simulink model "sampleModel1601_2"  (R2023a)
settings: Solver=VariableStepAuto  StartTime=0.0  StopTime=10.0  RelTol=1e-3
libraries: hdlsllib x2, simulink x1
settings Model: Creator=user1  LastModifiedBy=user1

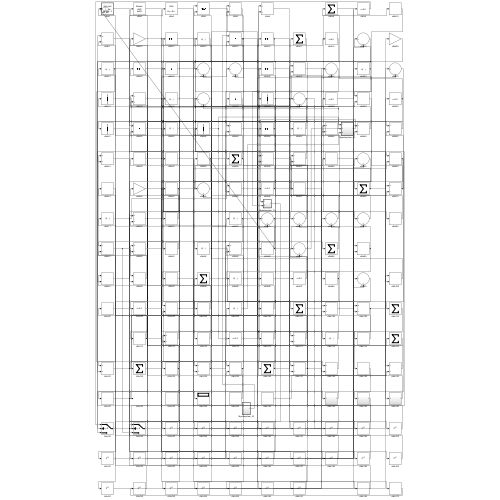
[thumbnail: Simulink's stored preview of the top-level diagram]
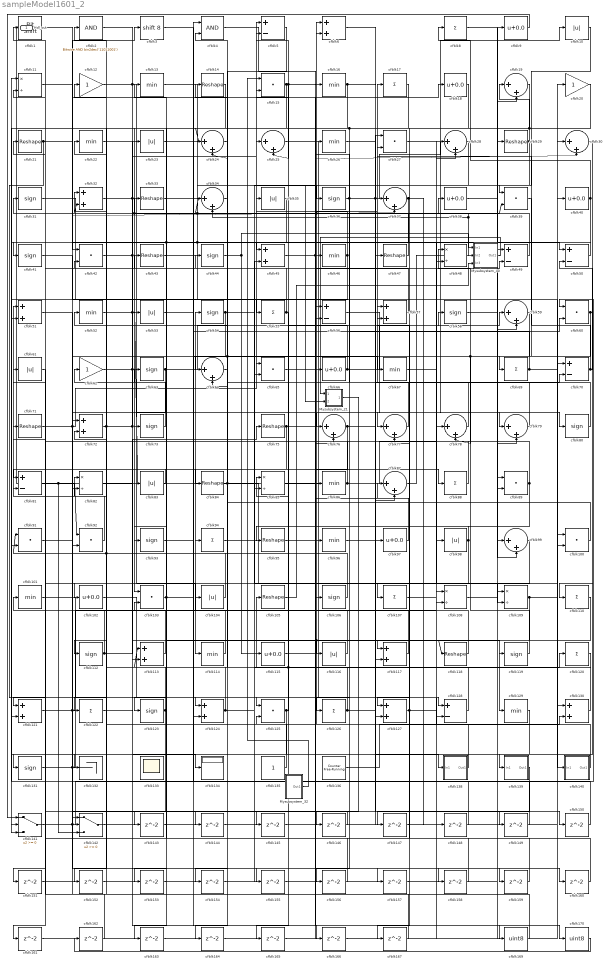
== system sampleModel1601_2 ==
  Mysubsystem_21 : Subsystem  TreatAsAtomicUnit=on  RTWFcnName=Mysubsystem_21
      settings: RTWFcnNameOpts=User specified  RTWFileNameOpts=Use function name
  Mysubsystem_32 : Subsystem  TreatAsAtomicUnit=on  RTWFcnName=Mysubsystem_32
      settings: RTWFcnNameOpts=User specified  RTWFileNameOpts=Use function name
  Mysubsystem_40 : Subsystem  TreatAsAtomicUnit=on  RTWFcnName=Mysubsystem_40
      settings: RTWFcnNameOpts=User specified  RTWFileNameOpts=Use function name
  cfblk1 : hdlsllib/Logic and Bit Operations/Bit Shift  mode=Shift Left Logical  N=0
  cfblk{10,23,35,53,61,83,98,104,116} (9 alike) : Abs  OutDataTypeStr=uint8  SaturateOnIntegerOverflow=off
  cfblk{15,27,39,42,60,65,89,91..92,100,103,125} (12 alike) : DotProduct  OutDataTypeStr=uint8
  cfblk{13,16,22,26,46,52,67,86,96,101,114,129} (12 alike) : MinMax  OutDataTypeStr=uint8
  cfblk{9,18,38,40,66,97,102,115} (8 alike) : Bias  Bias=0.0  SaturateOnIntegerOverflow=off
  cfblk{14,21,29,33,43,47,71,75,84,95,105,118} (12 alike) : Reshape
  cfblk{31,36,41,44,54,58,63,73,80,93,106,112,119,123,131} (15 alike) : Signum
  cfblk{8,17,55,69,88,94,107,110,120,122,126} (11 alike) : Sum  Inputs=+  OutDataTypeStr=uint8
  cfblk{11,48,82,85,108..109} (6 alike) : Product  Inputs=*/  OutDataTypeStr=uint8  RndMeth=Zero  SaturateOnIntegerOverflow=on
  cfblk{6,32,45,51,57,72,113,117,121,124,127,130} (12 alike) : Sum  OutDataTypeStr=uint8
  cfblk12 : Gain  OutDataTypeStr=uint8
  cfblk{5,49..50,56,70,81,128} (7 alike) : Sum  Inputs=+-  OutDataTypeStr=uint8
  cfblk132 : Terminator
  cfblk133 : Scope
      settings: Floating=on
  cfblk134 : Display
  cfblk135 : Constant  OutDataTypeStr=uint8  SampleTime=-1
  cfblk136 : hdlsllib/Sources/Counter Free-Running  NumBits=16  tsamp=-1
  cfblk138 : Subsystem
      settings: LibrarySourceBlock=|
      | hdlsllib/Ports &
      | Subsystems/Subsystem
  cfblk139 : Subsystem
      settings: LibrarySourceBlock=|
      | hdlsllib/Ports &
      | Subsystems/Subsystem
  cfblk140 : Subsystem
      settings: LibrarySourceBlock=|
      | hdlsllib/Ports &
      | Subsystems/Subsystem
  cfblk141 : Switch  OutDataTypeStr=uint8  SaturateOnIntegerOverflow=off  InputSameDT=off
  cfblk142 : Switch  OutDataTypeStr=uint8  SaturateOnIntegerOverflow=off  InputSameDT=off
  cfblk{143..167} (25 alike) : Delay  SampleTime=1
  cfblk169 : DataTypeConversion  OutDataTypeStr=uint8  SaturateOnIntegerOverflow=off  RndMeth=Floor
  cfblk170 : DataTypeConversion  OutDataTypeStr=uint8  SaturateOnIntegerOverflow=off  RndMeth=Floor
  cfblk{19,24..25,28,30,34,37,59,64,76..79,87,99} (15 alike) : Sum  Inputs=|++  OutDataTypeStr=uint8
  cfblk2 : simulink/Logic and Bit Operations/Bitwise Operator  logicop=AND  UseBitMask=on  BitMask=bin2dec('11011001')  BitMaskRealWorld=Stored Integer
      settings: LibrarySourceBlock=|
      | hdlsllib/Logic and Bit
      | Operations/Bitwise
      | Operator
  cfblk20 : Gain  OutDataTypeStr=uint8
  cfblk3 : ArithShift  BitShiftNumber=8
  cfblk4 : Logic  AllPortsSameDT=off  OutDataTypeStr=boolean
  cfblk62 : Gain  OutDataTypeStr=uint8
  Hdl_out : Outport  OutDataTypeStr=uint8
  wires:
  cfblk80/1 -> cfblk5/1
  cfblk92/1 -> cfblk51/1
  cfblk117/1 -> cfblk54/1
  cfblk60/1 -> cfblk131/1, cfblk113/2
  cfblk120/1 -> cfblk62/1
  cfblk104/1 -> cfblk91/1, cfblk72/2
  cfblk19/1 -> cfblk103/1
  cfblk32/1 -> cfblk77/1, cfblk134/1
  cfblk27/1 -> cfblk79/1
  cfblk141/1 -> cfblk60/1, cfblk160/1
  cfblk77/1 -> cfblk17/1
  cfblk116/1 -> cfblk61/1
  cfblk21/1 -> cfblk128/1, cfblk3/1
  cfblk30/1 -> cfblk110/1
  cfblk25/1 -> cfblk128/2
  cfblk10/1 -> cfblk39/1
  cfblk138/1(Out1) -> cfblk6/1
  cfblk56/1 -> cfblk89/1
  cfblk37/1 -> cfblk91/2, cfblk73/1, cfblk148/1
  cfblk47/1 -> cfblk6/2, cfblk34/1
  cfblk18/1 -> cfblk127/1
  cfblk63/1 -> cfblk58/1, cfblk92/2
  cfblk78/1 -> cfblk52/1
  cfblk66/1 -> cfblk59/1, cfblk5/2
  cfblk22/1 -> cfblk114/1
  cfblk12/1 -> cfblk76/1, cfblk50/1
  cfblk52/1 -> cfblk83/1, cfblk38/1
  cfblk13/1 -> cfblk100/2
  cfblk33/1 -> cfblk140/1(In1), cfblk98/1, cfblk39/2
  cfblk69/1 -> cfblk30/1, cfblk26/1
  cfblk115/1 -> cfblk66/1
  cfblk136/1 -> cfblk20/1
  cfblk31/1 -> cfblk53/1
  cfblk43/1 -> cfblk106/1
  cfblk20/1 -> cfblk51/2
  cfblk98/1 -> cfblk95/1, cfblk163/1
  cfblk29/1 -> cfblk19/1, cfblk24/1, cfblk65/2
  cfblk8/1 -> cfblk99/1
  cfblk130/1 -> cfblk105/1
  cfblk48/1 -> cfblk31/1, cfblk34/2
  cfblk15/1 -> cfblk25/2, cfblk169/1, cfblk123/1
  cfblk113/1 -> cfblk101/1
  cfblk44/1 -> Mysubsystem_40/1(In1), cfblk115/1
  cfblk101/1 -> cfblk124/1
  cfblk82/1 -> cfblk127/2
  cfblk72/1 -> cfblk23/1, cfblk158/1, cfblk122/1
  cfblk106/1 -> cfblk12/1
  cfblk23/1 -> cfblk36/1
  cfblk97/1 -> cfblk86/1
  cfblk142/1 -> cfblk108/1
  cfblk36/1 -> cfblk10/1, cfblk138/1(In1), cfblk156/1
  cfblk109/1 -> cfblk40/1, cfblk153/1
  cfblk85/1 -> cfblk37/1
  cfblk1/1 -> cfblk42/1
  cfblk58/1 -> cfblk99/2
  cfblk79/1 -> cfblk46/1
  cfblk102/1 -> cfblk125/1
  cfblk129/1 -> cfblk139/1(In1)
  cfblk81/1 -> cfblk92/1, cfblk142/3
  cfblk17/1 -> cfblk126/1, cfblk124/2
  cfblk50/1 -> cfblk41/1
  cfblk9/1 -> cfblk141/1
  cfblk89/1 -> cfblk57/1, cfblk167/1
  cfblk124/1 -> cfblk22/1, cfblk120/1
  cfblk61/1 -> cfblk121/1
  cfblk110/1 -> cfblk129/1
  cfblk75/1 -> cfblk117/1, cfblk164/1
  cfblk38/1 -> cfblk9/1
  cfblk62/1 -> cfblk80/1, cfblk159/1
  cfblk114/1 -> cfblk63/1
  cfblk64/1 -> cfblk14/1
  cfblk125/1 -> cfblk85/1, cfblk141/3
  cfblk40/1 -> cfblk93/1, cfblk152/1, cfblk8/1
  cfblk123/1 -> cfblk82/1, cfblk161/1
  cfblk59/1 -> cfblk82/2, cfblk84/1, cfblk78/2
  cfblk67/1 -> cfblk109/2
  cfblk107/1 -> cfblk28/1
  cfblk5/1 -> cfblk104/1
  cfblk83/1 -> cfblk81/1
  cfblk57/1 -> cfblk13/1
  cfblk39/1 -> cfblk69/1
  cfblk103/1 -> cfblk43/1, cfblk60/2
  cfblk119/1 -> cfblk48/1
  cfblk46/1 -> cfblk121/2, cfblk35/1
  cfblk35/1 -> cfblk102/1
  cfblk42/1 -> cfblk118/1, cfblk116/1, cfblk25/1
  cfblk54/1 -> cfblk64/1, cfblk107/1
  cfblk128/1 -> cfblk94/1
  cfblk91/1 -> cfblk16/1
  cfblk84/1 -> cfblk130/1, cfblk24/2
  cfblk73/1 -> cfblk32/1
  cfblk26/1 -> cfblk47/1
  cfblk4/1 -> cfblk96/1
  cfblk131/1 -> cfblk48/2, cfblk155/1
  cfblk11/1 -> cfblk45/1
  cfblk126/1 -> cfblk113/1, cfblk15/2, cfblk97/1
  cfblk96/1 -> cfblk70/2
  cfblk112/1 -> cfblk71/1, cfblk75/1
  cfblk45/1 -> cfblk30/2, cfblk49/2
  cfblk118/1 -> cfblk4/2
  cfblk14/1 -> cfblk141/2
  cfblk65/1 -> cfblk88/1
  cfblk135/1 -> cfblk42/2
  cfblk86/1 -> cfblk64/2, cfblk28/2, Hdl_out/1
  cfblk127/1 -> cfblk130/2, cfblk87/1
  cfblk121/1 -> cfblk56/1, cfblk37/2
  cfblk94/1 -> cfblk117/2
  cfblk16/1 -> cfblk132/1, cfblk149/1
  cfblk70/1 -> cfblk27/2, cfblk50/2
  cfblk95/1 -> cfblk18/1
  cfblk6/1 -> cfblk119/1
  cfblk108/1 -> cfblk29/1
  cfblk140/1(Out1) -> cfblk125/2
  cfblk76/1 -> cfblk112/1, cfblk87/2
  cfblk53/1 -> cfblk67/1
  cfblk49/1 -> cfblk33/1, cfblk32/2
  cfblk41/1 -> cfblk55/1
  cfblk71/1 -> cfblk65/1, cfblk146/1
  cfblk55/1 -> cfblk21/1, cfblk165/1
  cfblk88/1 -> cfblk11/2
  cfblk100/1 -> cfblk44/1
  cfblk143/1 -> cfblk56/2
  cfblk24/1 -> cfblk144/1
  cfblk144/1 -> cfblk27/1
  cfblk51/1 -> cfblk145/1
  cfblk145/1 -> cfblk79/2
  cfblk146/1 -> cfblk142/2
  cfblk139/1(Out1) -> cfblk147/1
  cfblk147/1 -> cfblk100/1
  cfblk148/1 -> cfblk11/1
  cfblk149/1 -> cfblk57/2
  cfblk93/1 -> cfblk150/1
  cfblk150/1 -> cfblk4/1
  cfblk99/1 -> cfblk151/1
  cfblk151/1 -> cfblk109/1
  cfblk152/1 -> cfblk85/2
  cfblk153/1 -> cfblk45/2
  cfblk34/1 -> cfblk154/1
  cfblk154/1 -> cfblk49/1
  cfblk155/1 -> cfblk59/2
  cfblk156/1 -> cfblk72/1
  cfblk122/1 -> cfblk157/1
  cfblk157/1 -> cfblk19/2
  cfblk158/1 -> cfblk77/2
  cfblk159/1 -> cfblk81/2
  cfblk160/1 -> cfblk103/2
  cfblk161/1 -> cfblk108/2
  cfblk162/1 -> cfblk142/1
  cfblk163/1 -> cfblk78/1
  cfblk164/1 -> cfblk76/2
  cfblk165/1 -> cfblk89/2
  cfblk3/1 -> cfblk166/1
  cfblk166/1 -> cfblk70/1
  cfblk167/1 -> cfblk1/1
  cfblk169/1 -> cfblk2/1
  cfblk2/1 -> cfblk170/1
  cfblk170/1 -> cfblk162/1
  cfblk28/1 -> Mysubsystem_21/2(In2)
  Mysubsystem_21/1(Out1) -> cfblk143/1
  Mysubsystem_32/1(Out1) -> cfblk15/1
  cfblk87/1 -> Mysubsystem_40/2(In2)
  cfblk105/1 -> Mysubsystem_40/3(In3)
  Mysubsystem_40/1(Out1) -> Mysubsystem_21/1(In1)

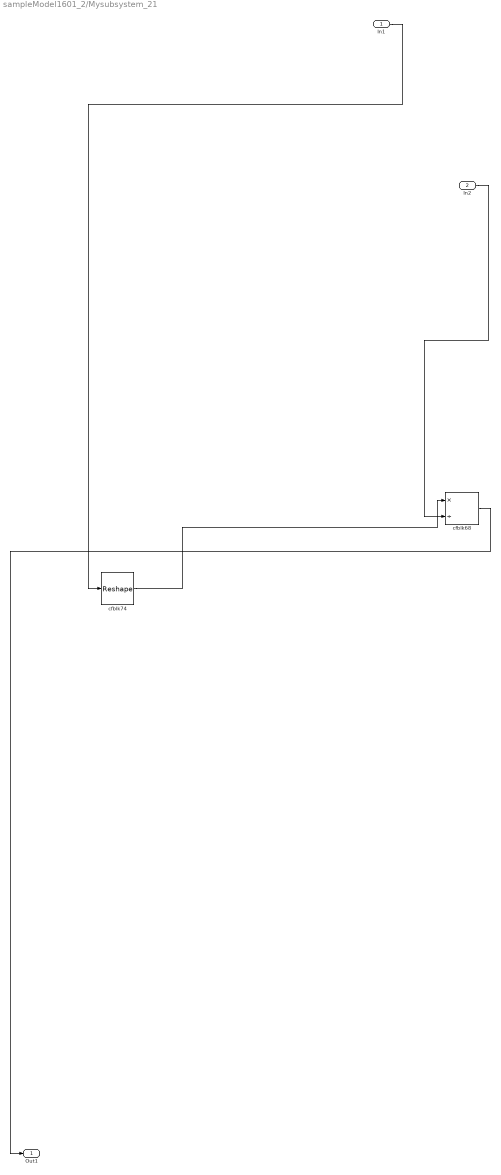
== system sampleModel1601_2/Mysubsystem_21 ==
  In1 : Inport
  In2 : Inport  Port=2
  cfblk68 : Product  Inputs=*/  RndMeth=Zero  SaturateOnIntegerOverflow=on
  cfblk74 : Reshape
  Out1 : Outport
  wires:
  cfblk74/1 -> cfblk68/1
  cfblk68/1 -> Out1/1
  In2/1 -> cfblk68/2
  In1/1 -> cfblk74/1

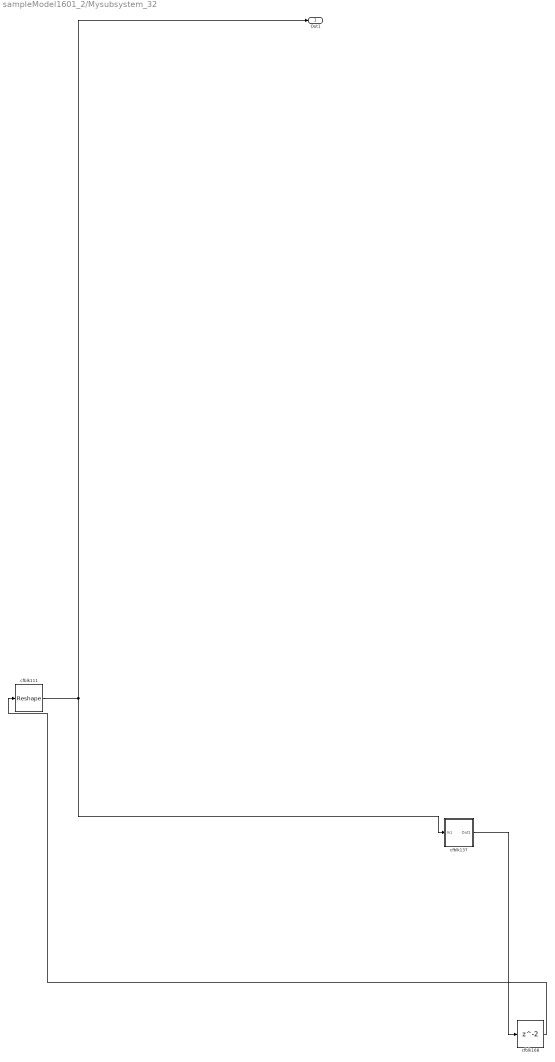
== system sampleModel1601_2/Mysubsystem_32 ==
  cfblk111 : Reshape
  cfblk137 : Subsystem
      settings: LibrarySourceBlock=|
      | hdlsllib/Ports &
      | Subsystems/Subsystem
  cfblk168 : Delay  SampleTime=1
  Out1 : Outport
  wires:
  cfblk137/1(Out1) -> cfblk168/1
  cfblk111/1 -> Out1/1, cfblk137/1(In1)
  cfblk168/1 -> cfblk111/1

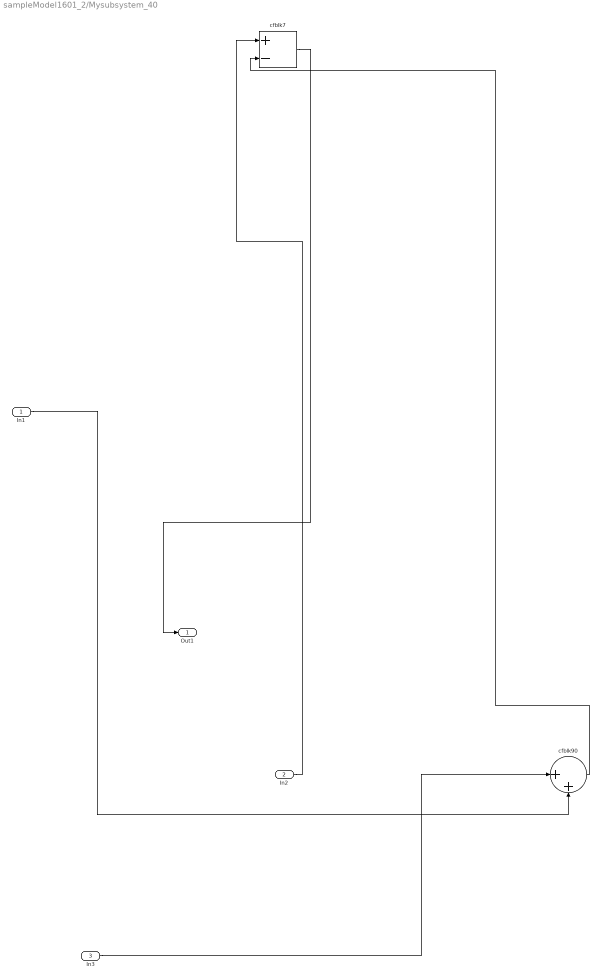
== system sampleModel1601_2/Mysubsystem_40 ==
  In1 : Inport
  In2 : Inport  Port=2
  In3 : Inport  Port=3
  cfblk7 : Sum  Inputs=+-
  cfblk90 : Sum  Inputs=|++
  Out1 : Outport
  wires:
  cfblk90/1 -> cfblk7/2
  In1/1 -> cfblk90/2
  In2/1 -> cfblk7/1
  cfblk7/1 -> Out1/1
  In3/1 -> cfblk90/1

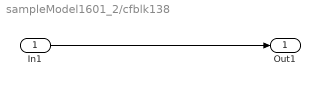
== system sampleModel1601_2/cfblk138 ==
  In1 : Inport
  Out1 : Outport
  wires:
  In1/1 -> Out1/1

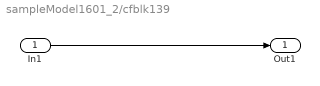
== system sampleModel1601_2/cfblk139 ==
  In1 : Inport
  Out1 : Outport
  wires:
  In1/1 -> Out1/1

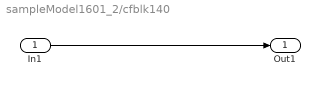
== system sampleModel1601_2/cfblk140 ==
  In1 : Inport
  Out1 : Outport
  wires:
  In1/1 -> Out1/1

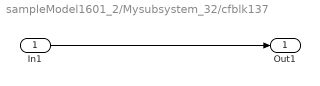
== system sampleModel1601_2/Mysubsystem_32/cfblk137 ==
  In1 : Inport
  Out1 : Outport
  wires:
  In1/1 -> Out1/1
